simulink model "motor_control"  (R2024b)
settings: Solver=VariableStepAuto  StartTime=0.0  StopTime=10.0  RelTol=1e-3
values from neighbouring files (symbols this model uses):
  K = 1.5    [motorSim_stepTest.m]
  Kp = 1.75    [motorSim_stepTest.m]
  sigma = 14    [motorSim_stepTest.m]
libraries: simulink x1
settings Model: Creator=rtgai  LastModifiedBy=rtgai

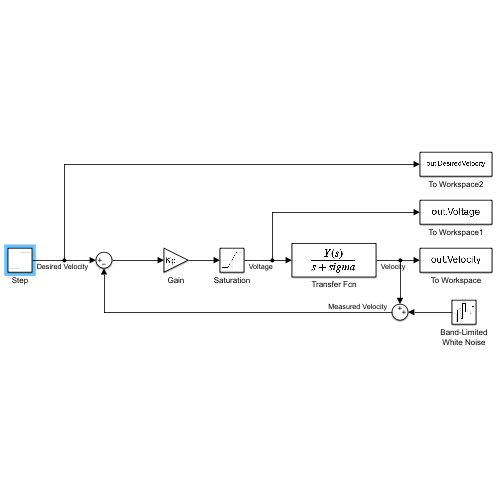
[thumbnail: Simulink's stored preview of the top-level diagram]
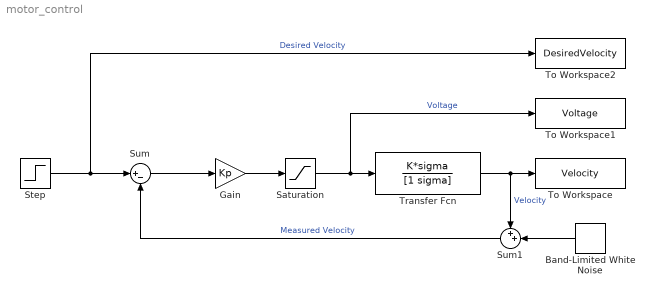
== system motor_control ==
  Band-Limited White Noise : simulink/Sources/Band-Limited White Noise  Cov=[0.0001]  Ts=0.01  seed=[23341]
  Gain : Gain  Gain=Kp
  Saturation : Saturate  UpperLimit=7.5  LowerLimit=-7.5
  Step : Step  After=3  SampleTime=0
  Sum : Sum  Inputs=|+-
  Sum1 : Sum  Inputs=++|
  To Workspace : ToWorkspace  VariableName=Velocity  SaveFormat=Timeseries  SampleTime=-1
  To Workspace1 : ToWorkspace  VariableName=Voltage  SaveFormat=Timeseries  SampleTime=-1
  To Workspace2 : ToWorkspace  VariableName=DesiredVelocity  SaveFormat=Timeseries  SampleTime=-1
  Transfer Fcn : TransferFcn  Numerator=K*sigma  Denominator=[1 sigma]
  wires:
  Step/1 -> To Workspace2/1, Sum/1  "Desired Velocity"
  Sum/1 -> Gain/1
  Gain/1 -> Saturation/1
  Saturation/1 -> To Workspace1/1, Transfer Fcn/1  "Voltage"
  Transfer Fcn/1 -> To Workspace/1, Sum1/1  "Velocity"
  Band-Limited White Noise/1 -> Sum1/2
  Sum1/1 -> Sum/2  "Measured Velocity"
